simulink model "four_tanks_baseline"  (Simulink 7.5)
settings: Solver=ode45  StartTime=0.0  StopTime=8000  MaxStep=.25  RelTol=1e-3
model workspace (MAT data in the model file):
  gamma_1 : Simulink.Parameter (value not decoded)
  gamma_2 : Simulink.Parameter (value not decoded)
  a1 : Simulink.Parameter (value not decoded)
  a2 : Simulink.Parameter (value not decoded)
  a3 : Simulink.Parameter (value not decoded)
  a4 : Simulink.Parameter (value not decoded)
  g : Simulink.Parameter (value not decoded)
  A_1 : Simulink.Parameter (value not decoded)
  A_2 : Simulink.Parameter (value not decoded)
  A_3 : Simulink.Parameter (value not decoded)
  A_4 : Simulink.Parameter (value not decoded)
  x1o : Simulink.Parameter (value not decoded)
  x2o : Simulink.Parameter (value not decoded)
  x3o : Simulink.Parameter (value not decoded)
  x4o : Simulink.Parameter (value not decoded)
  x1_max : Simulink.Parameter (value not decoded)
  x2_max : Simulink.Parameter (value not decoded)
  x3_max : Simulink.Parameter (value not decoded)
  x4_max : Simulink.Parameter (value not decoded)
  u1_max : Simulink.Parameter (value not decoded)
  u2_max : Simulink.Parameter (value not decoded)
  x1f : Simulink.Parameter (value not decoded)
  x2f : Simulink.Parameter (value not decoded)
settings Model: Creator=Administrator  LastModifiedBy=jporter
settings DebuggingCC: StrictBusMsg=Warning

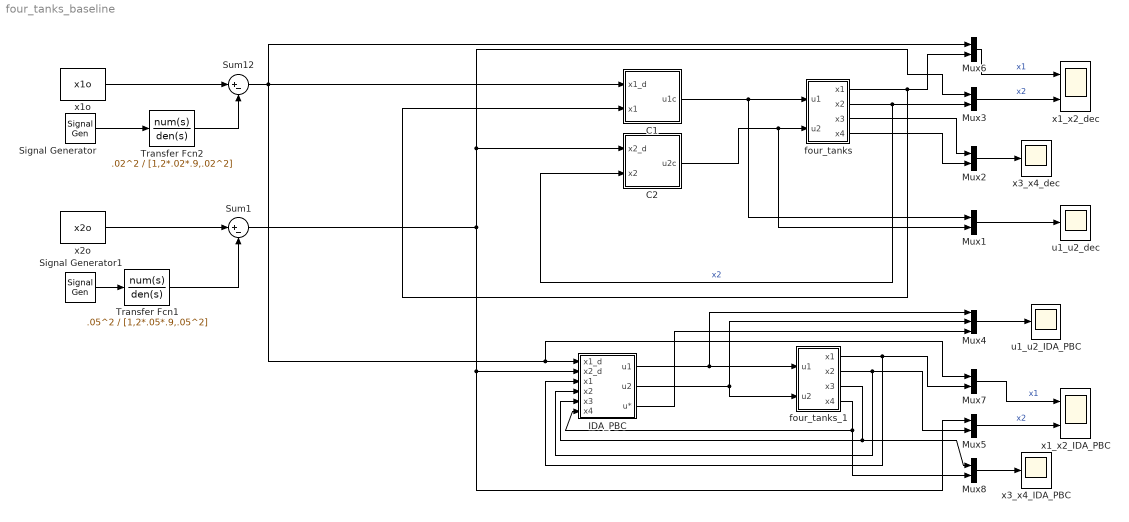
== system four_tanks_baseline ==
  C1 : Subsystem  mask{K=1.5, Ti=110, u1_max=100, gamma_1=gamma_1, gamma_2=gamma_2, x1o=x1o, x2o=x2o, a1=a1, a2=a2, g=g}
      mask prompts: u1_max "u1_max (ml/sec)"
      mask init:
      | L12 = [gamma_1, (1-gamma_2);
      |     (1-gamma_1),gamma_2];
      | us=inv(L12)*[a1*sqrt(2*g*x1o);a2*sqrt(2*g*x2o)];
      | xIo1=us(1)/K
  C2 : Subsystem  mask{K=-.12, Ti=220, u1_max=100, gamma_1=gamma_1, gamma_2=gamma_2, x1o=x1o, x2o=x2o, a1=a1, a2=a2, g=g}
      mask prompts: u1_max "u2_max (ml/sec)"
      mask init:
      | L12 = [gamma_1, (1-gamma_2);
      |     (1-gamma_1),gamma_2];
      | us=inv(L12)*[a1*sqrt(2*g*x1o);a2*sqrt(2*g*x2o)];
      | xIo2=us(2)/K
  IDA_PBC : Subsystem  mask{k1=.2, k2=.2, A_1=A_1, A_2=A_2, A_3=A_3, A_4=A_4, a1=a1, a2=a2, a3=a3, a4=a4, gamma_1=gamma_1, gamma_2=gamma_2, u1_max=u1_max, u2_max=u2_max, g=g}
      mask prompts: gamma_1 "gamma_1 in [0,1]"; gamma_2 "gamma_2 in [0,1]"; g "g (cm/s^2)"
      mask init:
      | k3=2*k1*A_3/(4*A_1);
      | k4=2*k2*A_4/(4*A_2);
      | kI1=0.1*(4-(k1/k3));
      | kI2=0.1*(4-(k2/k4));
      | JmR=[-1/(k1*A_1),0,1/(k3*A_1),0,0,0;
      |    0,-1/(k2*A_2),0,1/(k4*A_2),0,0;
      |    0,0,-1/(k3*A_3),0,0,0;
      |    0,0,0,-1/(k4*A_4),0,0;
      |    kI1/k1,0,0,0,-kI1/k1,0;
      |    0,kI2/k2,0,0,0,-kI2/k2];
      | eig(JmR)
      | P=[gamma_1*k1,(1-gamma_1)*k2,0,(1-gamma_1)*k4,gamma_1*k1,(1-gamma_1)*k2;
      |    (1-gamma_2)*k1,gamma_2*k2,(1-gamma_2)*k3,0,(1-gamma_2)*k1,gamma_2*k2];
      | L12=[gamma_1,(1-gamma_2);
      |     (1-gamma_1),gamma_2];
      | L34=[0,(1-gamma_2);
      |     (1-gamma_1),0];
      | Q=eye(2);
      | K=Q*P;
  Mux{1..3,5..8} (7 alike) : Mux  Inputs=2
  Mux4 : Mux  Inputs=[1,1,2]
  Signal Generator : SignalGenerator  WaveForm=square  Amplitude=x1f-x1o  Frequency=1/8000
  Signal Generator1 : SignalGenerator  WaveForm=square  Amplitude=x2f-x2o+.001  Frequency=1/8000
  Sum1 : Sum  Inputs=|+-  OutDataType=fixdt(1, 16)  OutScaling=2^0
  Sum12 : Sum  Inputs=|+-  OutDataType=fixdt(1, 16)  OutScaling=2^0
  Transfer Fcn1 : TransferFcn  Numerator=.05^2  Denominator=[1,2*.05*.9,.05^2]
  Transfer Fcn2 : TransferFcn  Numerator=.02^2  Denominator=[1,2*.02*.9,.02^2]
  four_tanks : Subsystem  mask{x1o=x1o, x2o=x2o, x3o=x3o, x4o=x4o, x1_max=x1_max, x2_max=x2_max, x3_max=x3_max, x4_max=x4_max, u1_max=100, u2_max=100, a1=a1, a2=a2, a3=a3, a4=a4, A_1=A_1, A_2=A_2, A_3=A_3, A_4=A_4, gamma_1=gamma_1, gamma_2=gamma_2, g=g}
      mask prompts: x1o "x1o (cm)"; x2o "x2o (cm)"; x3o "x3o (cm)"; x4o "x4o (cm)"; x1_max "x1_max (cm)"; x2_max "x2_max (cm)"; x3_max "x3_max (cm)"; x4_max "x4_max (cm)"; u1_max "u1_max (ml/s)"; u2_max "u2_max (ml/s)"; a1 "a1 (cm2)"; a2 "a2 (cm2)"; a3 "a3 (cm2)"; a4 "a4 (cm2)"; A_1 "A_1 (cm2)"; A_2 "A_2 (cm2)"; A_3 "A_3 (cm2)"; A_4 "A_4 (cm2)"; gamma_1 "gamma_1 in [0,1]"; gamma_2 "gamma_2 in [0,1]"; g "g (cm/s2)"
  four_tanks_1 : Subsystem  mask{x1o=x1o, x2o=x2o, x3o=x3o, x4o=x4o, x1_max=x1_max, x2_max=x2_max, x3_max=x3_max, x4_max=x4_max, u1_max=100, u2_max=100, a1=a1, a2=a2, a3=a3, a4=a4, A_1=A_1, A_2=A_2, A_3=A_3, A_4=A_4, gamma_1=gamma_1, gamma_2=gamma_2, g=g}
      mask prompts: x1o "x1o (cm)"; x2o "x2o (cm)"; x3o "x3o (cm)"; x4o "x4o (cm)"; x1_max "x1_max (cm)"; x2_max "x2_max (cm)"; x3_max "x3_max (cm)"; x4_max "x4_max (cm)"; u1_max "u1_max (ml/s)"; u2_max "u2_max (ml/s)"; a1 "a1 (cm2)"; a2 "a2 (cm2)"; a3 "a3 (cm2)"; a4 "a4 (cm2)"; A_1 "A_1 (cm2)"; A_2 "A_2 (cm2)"; A_3 "A_3 (cm2)"; A_4 "A_4 (cm2)"; gamma_1 "gamma_1 in [0,1]"; gamma_2 "gamma_2 in [0,1]"; g "g (cm/s2)"
  u1_u2_IDA_PBC : Scope
      settings: TimeRange=200  YMin=8.25  YMax=11  SampleInput=on  SampleTime=2
  u1_u2_dec : Scope
      settings: TimeRange=200  YMin=0  YMax=40  SaveName=ScopeData5  SampleInput=on  SampleTime=2
  x1_x2_IDA_PBC : Scope  NumInputPorts=2
      settings: YMin=7.5~7.5  YMax=17.5~17.5  SaveName=ScopeData2  SampleInput=on  SampleTime=2
  x1_x2_dec : Scope  NumInputPorts=2
      settings: YMin=1~2.5  YMax=15~15  SaveName=ScopeData6  SampleInput=on  SampleTime=2
  x1o : Constant  Value=x1o  OutDataType=fixdt(1, 16)  OutScaling=2^0
  x2o : Constant  Value=x2o  OutDataType=fixdt(1, 16)  OutScaling=2^0
  x3_x4_IDA_PBC : Scope
      settings: TimeRange=200  YMin=2  YMax=9.5  SaveName=ScopeData3  SampleInput=on  SampleTime=2
  x3_x4_dec : Scope
      settings: TimeRange=200  YMin=0  YMax=40  SampleInput=on  SampleTime=2
  wires:
  Signal Generator/1 -> Transfer Fcn2/1
  x1o/1 -> Sum12/1
  four_tanks/3(x3) -> Mux2/1
  four_tanks/4(x4) -> Mux2/2
  Mux1/1 -> u1_u2_dec/1
  Mux2/1 -> x3_x4_dec/1
  Sum12/1 -> IDA_PBC/1(x1_d), Mux7/1, Mux6/1, C1/1(x1_d)
  four_tanks/1(x1) -> C1/2(x1), Mux6/2
  four_tanks/2(x2) -> Mux3/2, C2/2(x2)  "x2"
  Transfer Fcn2/1 -> Sum12/2
  Mux3/1 -> x1_x2_dec/2  "x2"
  Mux6/1 -> x1_x2_dec/1  "x1"
  IDA_PBC/1(u1) -> four_tanks_1/1(u1), Mux4/1
  IDA_PBC/2(u2) -> four_tanks_1/2(u2), Mux4/2
  four_tanks_1/4(x4) -> IDA_PBC/6(x4), Mux8/2
  four_tanks_1/3(x3) -> IDA_PBC/5(x3), Mux8/1
  four_tanks_1/2(x2) -> IDA_PBC/4(x2), Mux5/2
  four_tanks_1/1(x1) -> IDA_PBC/3(x1), Mux7/2
  Mux4/1 -> u1_u2_IDA_PBC/1
  IDA_PBC/3(u*) -> Mux4/3
  Mux5/1 -> x1_x2_IDA_PBC/2  "x2"
  Mux7/1 -> x1_x2_IDA_PBC/1  "x1"
  Mux8/1 -> x3_x4_IDA_PBC/1
  Signal Generator1/1 -> Transfer Fcn1/1
  x2o/1 -> Sum1/1
  Transfer Fcn1/1 -> Sum1/2
  Sum1/1 -> IDA_PBC/2(x2_d), Mux5/1, Mux3/1, C2/1(x2_d)
  C1/1(u1c) -> four_tanks/1(u1), Mux1/1
  C2/1(u2c) -> four_tanks/2(u2), Mux1/2

== system four_tanks_baseline/C1 ==
  x1_d : Inport
  x1 : Inport  Port=2
  1/Ti : Gain  Gain=1/Ti  ParameterDataType=fixdt(1, 16)  ParameterScaling=2^0  OutDataType=fixdt(1, 16)  OutScaling=2^0
  Integrator1 : Integrator  InitialCondition=xIo1  LimitOutput=on  UpperSaturationLimit=u1_max/(abs(K))  LowerSaturationLimit=-u1_max/(abs(K))
  K : Gain  Gain=K  ParameterDataType=fixdt(1, 16)  ParameterScaling=2^0  OutDataType=fixdt(1, 16)  OutScaling=2^0
  SAT : Saturate  UpperLimit=u1_max  LowerLimit=0  OutDataType=fixdt(1, 16)  OutScaling=2^0
  Sum10 : Sum  Inputs=|+-  OutDataType=fixdt(1, 16)  OutScaling=2^0
  Sum11 : Sum  Inputs=++-  OutDataType=fixdt(1, 16)  OutScaling=2^0
  u1c : Outport
  wires:
  K/1 -> SAT/1
  Sum10/1 -> 1/Ti/1
  Sum11/1 -> K/1
  1/Ti/1 -> Integrator1/1
  Integrator1/1 -> Sum11/2
  x1_d/1 -> Sum11/1, Sum10/1
  SAT/1 -> u1c/1
  x1/1 -> Sum10/2, Sum11/3

== system four_tanks_baseline/C2 ==
  x2_d : Inport
  x2 : Inport  Port=2
  1/Ti : Gain  Gain=1/Ti  ParameterDataType=fixdt(1, 16)  ParameterScaling=2^0  OutDataType=fixdt(1, 16)  OutScaling=2^0
  Integrator1 : Integrator  InitialCondition=xIo2  LimitOutput=on  UpperSaturationLimit=u1_max/(abs(K))  LowerSaturationLimit=-u1_max/(abs(K))
  K : Gain  Gain=K  ParameterDataType=fixdt(1, 16)  ParameterScaling=2^0  OutDataType=fixdt(1, 16)  OutScaling=2^0
  SAT : Saturate  UpperLimit=u1_max  LowerLimit=0  OutDataType=fixdt(1, 16)  OutScaling=2^0
  Sum10 : Sum  Inputs=|+-  OutDataType=fixdt(1, 16)  OutScaling=2^0
  Sum11 : Sum  Inputs=++-  OutDataType=fixdt(1, 16)  OutScaling=2^0
  u2c : Outport
  wires:
  x2/1 -> Sum11/3, Sum10/2
  SAT/1 -> u2c/1
  x2_d/1 -> Sum10/1, Sum11/1
  Integrator1/1 -> Sum11/2
  1/Ti/1 -> Integrator1/1
  Sum11/1 -> K/1
  Sum10/1 -> 1/Ti/1
  K/1 -> SAT/1

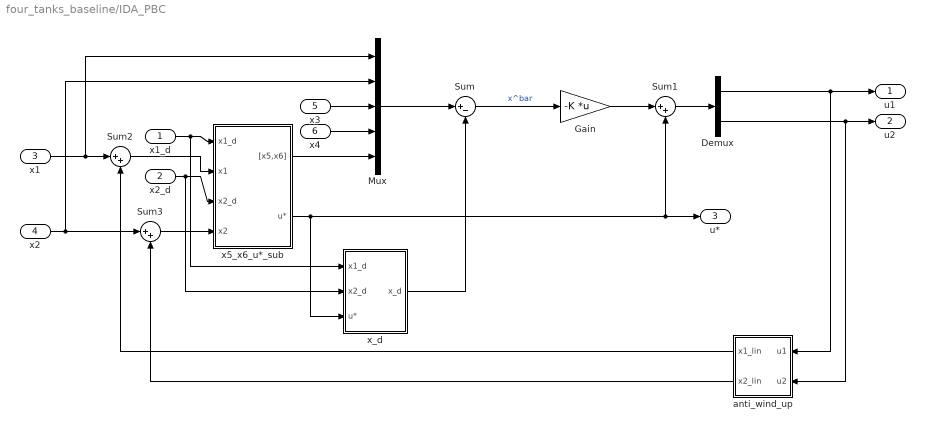
== system four_tanks_baseline/IDA_PBC ==
  x1_d : Inport
  x2_d : Inport  Port=2
  x1 : Inport  Port=3
  x2 : Inport  Port=4
  x3 : Inport  Port=5
  x4 : Inport  Port=6
  Demux : Demux  Outputs=2
  Gain : Gain  Gain=-K  Multiplication=Matrix(K*u)  ParameterDataType=fixdt(1, 16)  ParameterScaling=2^0  OutDataType=fixdt(1, 16)  OutScaling=2^0
  Mux : Mux  Inputs=[1,1,1,1,2]
  Sum : Sum  Inputs=|+-  OutDataType=fixdt(1, 16)  OutScaling=2^0
  Sum1 : Sum  Inputs=|++  OutDataType=fixdt(1, 16)  OutScaling=2^0
  Sum2 : Sum  Inputs=|++  OutDataType=fixdt(1, 16)  OutScaling=2^0
  Sum3 : Sum  Inputs=|++  OutDataType=fixdt(1, 16)  OutScaling=2^0
  anti_wind_up : Subsystem
  x5_x6_u*_sub : Subsystem
  x_d : Subsystem
  u1 : Outport
  u2 : Outport  Port=2
  u* : Outport  Port=3
  wires:
  x1_d/1 -> x5_x6_u*_sub/1(x1_d), x_d/1(x1_d)
  x1/1 -> Mux/1, Sum2/1
  x2_d/1 -> x5_x6_u*_sub/3(x2_d), x_d/2(x2_d)
  x2/1 -> Mux/2, Sum3/1
  x5_x6_u*_sub/1("[x5,x6]") -> Mux/5
  x3/1 -> Mux/3
  x4/1 -> Mux/4
  x5_x6_u*_sub/2(u*) -> x_d/3(u*), Sum1/2, u*/1
  Mux/1 -> Sum/1
  x_d/1(x_d) -> Sum/2
  Sum/1 -> Gain/1  "x^bar"
  Gain/1 -> Sum1/1
  Sum1/1 -> Demux/1
  Demux/1 -> u1/1, anti_wind_up/1(u1)
  Demux/2 -> u2/1, anti_wind_up/2(u2)
  anti_wind_up/1(x1_lin) -> Sum2/2
  Sum2/1 -> x5_x6_u*_sub/2(x1)
  Sum3/1 -> x5_x6_u*_sub/4(x2)
  anti_wind_up/2(x2_lin) -> Sum3/2

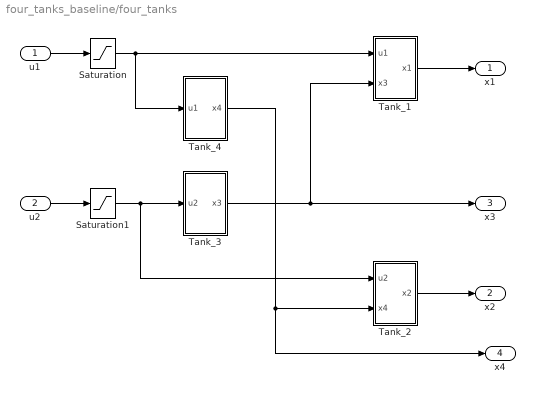
== system four_tanks_baseline/four_tanks ==
  u1 : Inport  OutDataType=fixdt(1, 16)  OutScaling=2^0
  u2 : Inport  Port=2  OutDataType=fixdt(1, 16)  OutScaling=2^0
  Saturation : Saturate  UpperLimit=u1_max  LowerLimit=0  OutDataType=fixdt(1, 16)  OutScaling=2^0
  Saturation1 : Saturate  UpperLimit=u2_max  LowerLimit=0  OutDataType=fixdt(1, 16)  OutScaling=2^0
  Tank_1 : Subsystem
  Tank_2 : Subsystem
  Tank_3 : Subsystem
  Tank_4 : Subsystem
  x1 : Outport  OutDataType=fixdt(1, 16)  OutScaling=2^0
  x2 : Outport  Port=2  OutDataType=fixdt(1, 16)  OutScaling=2^0
  x3 : Outport  Port=3  OutDataType=fixdt(1, 16)  OutScaling=2^0
  x4 : Outport  Port=4  OutDataType=fixdt(1, 16)  OutScaling=2^0
  wires:
  u1/1 -> Saturation/1
  Tank_1/1(x1) -> x1/1
  Tank_2/1(x2) -> x2/1
  u2/1 -> Saturation1/1
  Saturation/1 -> Tank_1/1(u1), Tank_4/1(u1)
  Saturation1/1 -> Tank_3/1(u2), Tank_2/1(u2)
  Tank_3/1(x3) -> Tank_1/2(x3), x3/1
  Tank_4/1(x4) -> Tank_2/2(x4), x4/1

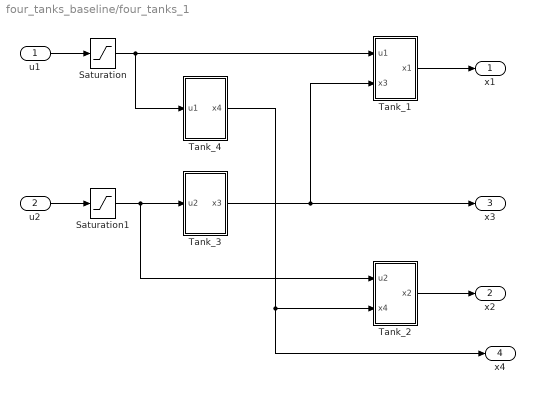
== system four_tanks_baseline/four_tanks_1 ==
  u1 : Inport  OutDataType=fixdt(1, 16)  OutScaling=2^0
  u2 : Inport  Port=2  OutDataType=fixdt(1, 16)  OutScaling=2^0
  Saturation : Saturate  UpperLimit=u1_max  LowerLimit=0  OutDataType=fixdt(1, 16)  OutScaling=2^0
  Saturation1 : Saturate  UpperLimit=u2_max  LowerLimit=0  OutDataType=fixdt(1, 16)  OutScaling=2^0
  Tank_1 : Subsystem
  Tank_2 : Subsystem
  Tank_3 : Subsystem
  Tank_4 : Subsystem
  x1 : Outport  OutDataType=fixdt(1, 16)  OutScaling=2^0
  x2 : Outport  Port=2  OutDataType=fixdt(1, 16)  OutScaling=2^0
  x3 : Outport  Port=3  OutDataType=fixdt(1, 16)  OutScaling=2^0
  x4 : Outport  Port=4  OutDataType=fixdt(1, 16)  OutScaling=2^0
  wires:
  Tank_4/1(x4) -> x4/1, Tank_2/2(x4)
  Tank_3/1(x3) -> x3/1, Tank_1/2(x3)
  Saturation1/1 -> Tank_2/1(u2), Tank_3/1(u2)
  Saturation/1 -> Tank_4/1(u1), Tank_1/1(u1)
  u2/1 -> Saturation1/1
  Tank_2/1(x2) -> x2/1
  Tank_1/1(x1) -> x1/1
  u1/1 -> Saturation/1

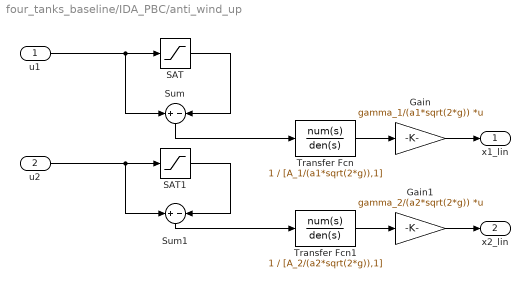
== system four_tanks_baseline/IDA_PBC/anti_wind_up ==
  u1 : Inport
  u2 : Inport  Port=2
  Gain : Gain  Gain=gamma_1/(a1*sqrt(2*g))  Multiplication=Matrix(K*u)  ParameterDataType=fixdt(1, 16)  ParameterScaling=2^0  OutDataType=fixdt(1, 16)  OutScaling=2^0
  Gain1 : Gain  Gain=gamma_2/(a2*sqrt(2*g))  Multiplication=Matrix(K*u)  ParameterDataType=fixdt(1, 16)  ParameterScaling=2^0  OutDataType=fixdt(1, 16)  OutScaling=2^0
  SAT : Saturate  UpperLimit=u1_max  LowerLimit=0  OutDataType=fixdt(1, 16)  OutScaling=2^0
  SAT1 : Saturate  UpperLimit=u1_max  LowerLimit=0  OutDataType=fixdt(1, 16)  OutScaling=2^0
  Sum : Sum  Inputs=+-  OutDataType=fixdt(1, 16)  OutScaling=2^0
  Sum1 : Sum  Inputs=+-  OutDataType=fixdt(1, 16)  OutScaling=2^0
  Transfer Fcn : TransferFcn  Numerator=1  Denominator=[A_1/(a1*sqrt(2*g)),1]
  Transfer Fcn1 : TransferFcn  Numerator=1  Denominator=[A_2/(a2*sqrt(2*g)),1]
  x1_lin : Outport
  x2_lin : Outport  Port=2
  wires:
  u1/1 -> SAT/1, Sum/1
  u2/1 -> SAT1/1, Sum1/1
  SAT/1 -> Sum/2
  SAT1/1 -> Sum1/2
  Sum/1 -> Transfer Fcn/1
  Transfer Fcn/1 -> Gain/1
  Gain/1 -> x1_lin/1
  Transfer Fcn1/1 -> Gain1/1
  Gain1/1 -> x2_lin/1
  Sum1/1 -> Transfer Fcn1/1

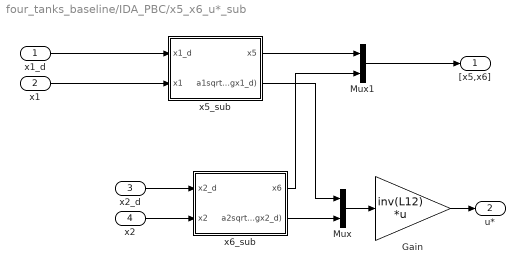
== system four_tanks_baseline/IDA_PBC/x5_x6_u*_sub ==
  x1_d : Inport
  x1 : Inport  Port=2
  x2_d : Inport  Port=3
  x2 : Inport  Port=4
  Gain : Gain  Gain=inv(L12)  Multiplication=Matrix(K*u)  ParameterDataType=fixdt(1, 16)  ParameterScaling=2^0  OutDataType=fixdt(1, 16)  OutScaling=2^0
  Mux : Mux  Inputs=2
  Mux1 : Mux  Inputs=2
  x5_sub : Subsystem
  x6_sub : Subsystem
  "[x5,x6]" : Outport
  u* : Outport  Port=2
  wires:
  x5_sub/2(a1sqrt(2gx1_d)) -> Mux/1
  x6_sub/2(a2sqrt(2gx2_d)) -> Mux/2
  Mux/1 -> Gain/1
  x5_sub/1(x5) -> Mux1/1
  x6_sub/1(x6) -> Mux1/2
  x1_d/1 -> x5_sub/1(x1_d)
  Mux1/1 -> "[x5,x6]"/1
  x1/1 -> x5_sub/2(x1)
  x2_d/1 -> x6_sub/1(x2_d)
  x2/1 -> x6_sub/2(x2)
  Gain/1 -> u*/1

== system four_tanks_baseline/IDA_PBC/x_d ==
  x1_d : Inport
  x2_d : Inport  Port=2
  u* : Inport  Port=3
  Mux1 : Mux  Inputs=[1,1,2,2]
  gen_x3d_x4d : Subsystem
  x5d_x6d : Constant  Value=[0,0]  OutDataType=fixdt(1, 16)  OutScaling=2^0
  x_d : Outport
  wires:
  x5d_x6d/1 -> Mux1/4
  gen_x3d_x4d/1("[x3d,x4d]") -> Mux1/3
  x1_d/1 -> Mux1/1
  x2_d/1 -> Mux1/2
  Mux1/1 -> x_d/1
  u*/1 -> gen_x3d_x4d/1(u*)

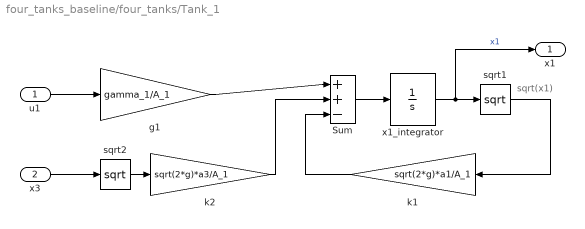
== system four_tanks_baseline/four_tanks/Tank_1 ==
  note: sqrt(x1)
  u1 : Inport
  x3 : Inport  Port=2
  Sum : Sum  Inputs=|++-  OutDataType=fixdt(1, 16)  OutScaling=2^0
  g1 : Gain  Gain=gamma_1/A_1  ParameterDataType=fixdt(1, 16)  ParameterScaling=2^0  OutDataType=fixdt(1, 16)  OutScaling=2^0
  k1 : Gain  Gain=sqrt(2*g)*a1/A_1  ParameterDataType=fixdt(1, 16)  ParameterScaling=2^0  OutDataType=fixdt(1, 16)  OutScaling=2^0
  k2 : Gain  Gain=sqrt(2*g)*a3/A_1  ParameterDataType=fixdt(1, 16)  ParameterScaling=2^0  OutDataType=fixdt(1, 16)  OutScaling=2^0
  sqrt1 : Math  Operator=sqrt  OutDataType=fixdt(1, 16)  OutScaling=2^0  SaturateOnIntegerOverflow=on
  sqrt2 : Math  Operator=sqrt  OutDataType=fixdt(1, 16)  OutScaling=2^0  SaturateOnIntegerOverflow=on
  x1_integrator : Integrator  InitialCondition=x1o  LimitOutput=on  UpperSaturationLimit=x1_max  LowerSaturationLimit=0
  x1 : Outport
  wires:
  g1/1 -> Sum/1
  x1_integrator/1 -> sqrt1/1, x1/1  "x1"
  sqrt1/1 -> k1/1
  k1/1 -> Sum/3
  Sum/1 -> x1_integrator/1
  u1/1 -> g1/1
  x3/1 -> sqrt2/1
  sqrt2/1 -> k2/1
  k2/1 -> Sum/2

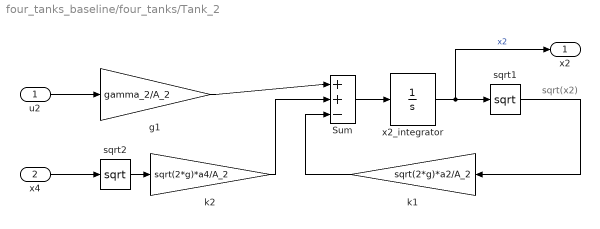
== system four_tanks_baseline/four_tanks/Tank_2 ==
  note: sqrt(x2)
  u2 : Inport
  x4 : Inport  Port=2
  Sum : Sum  Inputs=|++-  OutDataType=fixdt(1, 16)  OutScaling=2^0
  g1 : Gain  Gain=gamma_2/A_2  ParameterDataType=fixdt(1, 16)  ParameterScaling=2^0  OutDataType=fixdt(1, 16)  OutScaling=2^0
  k1 : Gain  Gain=sqrt(2*g)*a2/A_2  ParameterDataType=fixdt(1, 16)  ParameterScaling=2^0  OutDataType=fixdt(1, 16)  OutScaling=2^0
  k2 : Gain  Gain=sqrt(2*g)*a4/A_2  ParameterDataType=fixdt(1, 16)  ParameterScaling=2^0  OutDataType=fixdt(1, 16)  OutScaling=2^0
  sqrt1 : Math  Operator=sqrt  OutDataType=fixdt(1, 16)  OutScaling=2^0  SaturateOnIntegerOverflow=on
  sqrt2 : Math  Operator=sqrt  OutDataType=fixdt(1, 16)  OutScaling=2^0  SaturateOnIntegerOverflow=on
  x2_integrator : Integrator  InitialCondition=x2o  LimitOutput=on  UpperSaturationLimit=x2_max  LowerSaturationLimit=0
  x2 : Outport
  wires:
  k2/1 -> Sum/2
  sqrt2/1 -> k2/1
  x4/1 -> sqrt2/1
  u2/1 -> g1/1
  Sum/1 -> x2_integrator/1
  k1/1 -> Sum/3
  sqrt1/1 -> k1/1
  x2_integrator/1 -> x2/1, sqrt1/1  "x2"
  g1/1 -> Sum/1

== system four_tanks_baseline/four_tanks/Tank_3 ==
  note: sqrt(x3)
  u2 : Inport
  Sum : Sum  Inputs=|+-  OutDataType=fixdt(1, 16)  OutScaling=2^0
  g1 : Gain  Gain=(1-gamma_2)/A_3  ParameterDataType=fixdt(1, 16)  ParameterScaling=2^0  OutDataType=fixdt(1, 16)  OutScaling=2^0
  k1 : Gain  Gain=sqrt(2*g)*a3/A_3  ParameterDataType=fixdt(1, 16)  ParameterScaling=2^0  OutDataType=fixdt(1, 16)  OutScaling=2^0
  sqrt1 : Math  Operator=sqrt  OutDataType=fixdt(1, 16)  OutScaling=2^0  SaturateOnIntegerOverflow=on
  x3_integrator : Integrator  InitialCondition=x3o  LimitOutput=on  UpperSaturationLimit=x3_max  LowerSaturationLimit=0
  x3 : Outport
  wires:
  g1/1 -> Sum/1
  x3_integrator/1 -> sqrt1/1, x3/1  "x3"
  sqrt1/1 -> k1/1
  Sum/1 -> x3_integrator/1
  u2/1 -> g1/1
  k1/1 -> Sum/2

== system four_tanks_baseline/four_tanks/Tank_4 ==
  note: sqrt(x4)
  u1 : Inport
  Sum : Sum  Inputs=|+-  OutDataType=fixdt(1, 16)  OutScaling=2^0
  g1 : Gain  Gain=(1-gamma_1)/A_4  ParameterDataType=fixdt(1, 16)  ParameterScaling=2^0  OutDataType=fixdt(1, 16)  OutScaling=2^0
  k1 : Gain  Gain=sqrt(2*g)*a4/A_4  ParameterDataType=fixdt(1, 16)  ParameterScaling=2^0  OutDataType=fixdt(1, 16)  OutScaling=2^0
  sqrt1 : Math  Operator=sqrt  OutDataType=fixdt(1, 16)  OutScaling=2^0  SaturateOnIntegerOverflow=on
  x4_integrator : Integrator  InitialCondition=x4o  LimitOutput=on  UpperSaturationLimit=x4_max  LowerSaturationLimit=0
  x4 : Outport
  wires:
  k1/1 -> Sum/2
  u1/1 -> g1/1
  Sum/1 -> x4_integrator/1
  sqrt1/1 -> k1/1
  x4_integrator/1 -> x4/1, sqrt1/1  "x4"
  g1/1 -> Sum/1

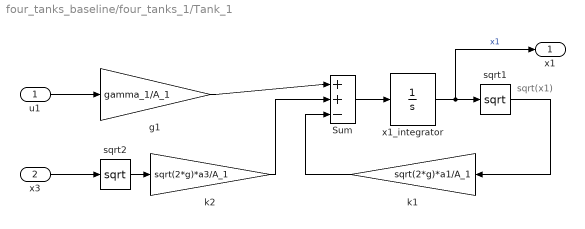
== system four_tanks_baseline/four_tanks_1/Tank_1 ==
  note: sqrt(x1)
  u1 : Inport
  x3 : Inport  Port=2
  Sum : Sum  Inputs=|++-  OutDataType=fixdt(1, 16)  OutScaling=2^0
  g1 : Gain  Gain=gamma_1/A_1  ParameterDataType=fixdt(1, 16)  ParameterScaling=2^0  OutDataType=fixdt(1, 16)  OutScaling=2^0
  k1 : Gain  Gain=sqrt(2*g)*a1/A_1  ParameterDataType=fixdt(1, 16)  ParameterScaling=2^0  OutDataType=fixdt(1, 16)  OutScaling=2^0
  k2 : Gain  Gain=sqrt(2*g)*a3/A_1  ParameterDataType=fixdt(1, 16)  ParameterScaling=2^0  OutDataType=fixdt(1, 16)  OutScaling=2^0
  sqrt1 : Math  Operator=sqrt  OutDataType=fixdt(1, 16)  OutScaling=2^0  SaturateOnIntegerOverflow=on
  sqrt2 : Math  Operator=sqrt  OutDataType=fixdt(1, 16)  OutScaling=2^0  SaturateOnIntegerOverflow=on
  x1_integrator : Integrator  InitialCondition=x1o  LimitOutput=on  UpperSaturationLimit=x1_max  LowerSaturationLimit=0
  x1 : Outport
  wires:
  k2/1 -> Sum/2
  sqrt2/1 -> k2/1
  x3/1 -> sqrt2/1
  u1/1 -> g1/1
  Sum/1 -> x1_integrator/1
  k1/1 -> Sum/3
  sqrt1/1 -> k1/1
  x1_integrator/1 -> x1/1, sqrt1/1  "x1"
  g1/1 -> Sum/1

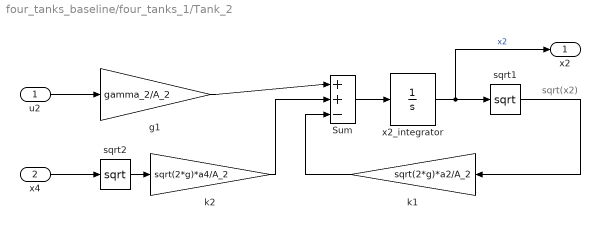
== system four_tanks_baseline/four_tanks_1/Tank_2 ==
  note: sqrt(x2)
  u2 : Inport
  x4 : Inport  Port=2
  Sum : Sum  Inputs=|++-  OutDataType=fixdt(1, 16)  OutScaling=2^0
  g1 : Gain  Gain=gamma_2/A_2  ParameterDataType=fixdt(1, 16)  ParameterScaling=2^0  OutDataType=fixdt(1, 16)  OutScaling=2^0
  k1 : Gain  Gain=sqrt(2*g)*a2/A_2  ParameterDataType=fixdt(1, 16)  ParameterScaling=2^0  OutDataType=fixdt(1, 16)  OutScaling=2^0
  k2 : Gain  Gain=sqrt(2*g)*a4/A_2  ParameterDataType=fixdt(1, 16)  ParameterScaling=2^0  OutDataType=fixdt(1, 16)  OutScaling=2^0
  sqrt1 : Math  Operator=sqrt  OutDataType=fixdt(1, 16)  OutScaling=2^0  SaturateOnIntegerOverflow=on
  sqrt2 : Math  Operator=sqrt  OutDataType=fixdt(1, 16)  OutScaling=2^0  SaturateOnIntegerOverflow=on
  x2_integrator : Integrator  InitialCondition=x2o  LimitOutput=on  UpperSaturationLimit=x2_max  LowerSaturationLimit=0
  x2 : Outport
  wires:
  g1/1 -> Sum/1
  x2_integrator/1 -> sqrt1/1, x2/1  "x2"
  sqrt1/1 -> k1/1
  k1/1 -> Sum/3
  Sum/1 -> x2_integrator/1
  u2/1 -> g1/1
  x4/1 -> sqrt2/1
  sqrt2/1 -> k2/1
  k2/1 -> Sum/2

== system four_tanks_baseline/four_tanks_1/Tank_3 ==
  note: sqrt(x3)
  u2 : Inport
  Sum : Sum  Inputs=|+-  OutDataType=fixdt(1, 16)  OutScaling=2^0
  g1 : Gain  Gain=(1-gamma_2)/A_3  ParameterDataType=fixdt(1, 16)  ParameterScaling=2^0  OutDataType=fixdt(1, 16)  OutScaling=2^0
  k1 : Gain  Gain=sqrt(2*g)*a3/A_3  ParameterDataType=fixdt(1, 16)  ParameterScaling=2^0  OutDataType=fixdt(1, 16)  OutScaling=2^0
  sqrt1 : Math  Operator=sqrt  OutDataType=fixdt(1, 16)  OutScaling=2^0  SaturateOnIntegerOverflow=on
  x3_integrator : Integrator  InitialCondition=x3o  LimitOutput=on  UpperSaturationLimit=x3_max  LowerSaturationLimit=0
  x3 : Outport
  wires:
  k1/1 -> Sum/2
  u2/1 -> g1/1
  Sum/1 -> x3_integrator/1
  sqrt1/1 -> k1/1
  x3_integrator/1 -> x3/1, sqrt1/1  "x3"
  g1/1 -> Sum/1

== system four_tanks_baseline/four_tanks_1/Tank_4 ==
  note: sqrt(x4)
  u1 : Inport
  Sum : Sum  Inputs=|+-  OutDataType=fixdt(1, 16)  OutScaling=2^0
  g1 : Gain  Gain=(1-gamma_1)/A_4  ParameterDataType=fixdt(1, 16)  ParameterScaling=2^0  OutDataType=fixdt(1, 16)  OutScaling=2^0
  k1 : Gain  Gain=sqrt(2*g)*a4/A_4  ParameterDataType=fixdt(1, 16)  ParameterScaling=2^0  OutDataType=fixdt(1, 16)  OutScaling=2^0
  sqrt1 : Math  Operator=sqrt  OutDataType=fixdt(1, 16)  OutScaling=2^0  SaturateOnIntegerOverflow=on
  x4_integrator : Integrator  InitialCondition=x4o  LimitOutput=on  UpperSaturationLimit=x4_max  LowerSaturationLimit=0
  x4 : Outport
  wires:
  g1/1 -> Sum/1
  x4_integrator/1 -> sqrt1/1, x4/1  "x4"
  sqrt1/1 -> k1/1
  Sum/1 -> x4_integrator/1
  u1/1 -> g1/1
  k1/1 -> Sum/2

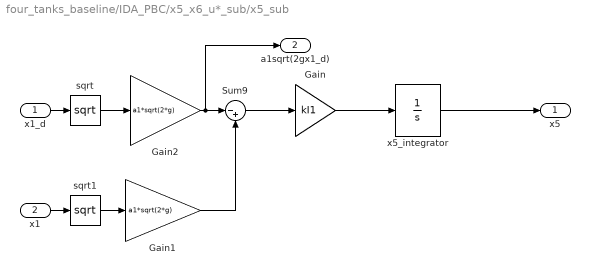
== system four_tanks_baseline/IDA_PBC/x5_x6_u*_sub/x5_sub ==
  x1_d : Inport
  x1 : Inport  Port=2
  Gain : Gain  Gain=kI1  ParameterDataType=fixdt(1, 16)  ParameterScaling=2^0  OutDataType=fixdt(1, 16)  OutScaling=2^0
  Gain1 : Gain  Gain=a1*sqrt(2*g)  ParameterDataType=fixdt(1, 16)  ParameterScaling=2^0  OutDataType=fixdt(1, 16)  OutScaling=2^0
  Gain2 : Gain  Gain=a1*sqrt(2*g)  ParameterDataType=fixdt(1, 16)  ParameterScaling=2^0  OutDataType=fixdt(1, 16)  OutScaling=2^0
  Sum9 : Sum  Inputs=|-+  OutDataType=fixdt(1, 16)  OutScaling=2^0
  sqrt : Math  Operator=sqrt  OutDataType=fixdt(1, 16)  OutScaling=2^0  SaturateOnIntegerOverflow=on
  sqrt1 : Math  Operator=sqrt  OutDataType=fixdt(1, 16)  OutScaling=2^0  SaturateOnIntegerOverflow=on
  x5_integrator : Integrator  UpperSaturationLimit=.1*sqrt(2*g*100)  LowerSaturationLimit=-.1*sqrt(2*g*100)
  x5 : Outport
  a1sqrt(2gx1_d) : Outport  Port=2
  wires:
  sqrt/1 -> Gain2/1
  sqrt1/1 -> Gain1/1
  Sum9/1 -> Gain/1
  x1_d/1 -> sqrt/1
  x5_integrator/1 -> x5/1
  x1/1 -> sqrt1/1
  Gain1/1 -> Sum9/2
  Gain2/1 -> Sum9/1, a1sqrt(2gx1_d)/1
  Gain/1 -> x5_integrator/1

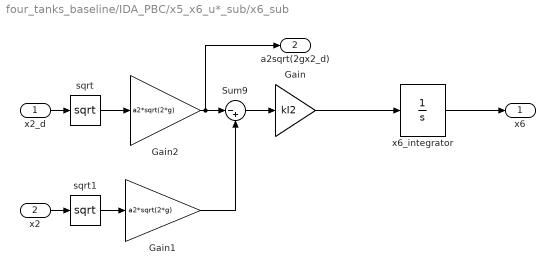
== system four_tanks_baseline/IDA_PBC/x5_x6_u*_sub/x6_sub ==
  x2_d : Inport
  x2 : Inport  Port=2
  Gain : Gain  Gain=kI2  ParameterDataType=fixdt(1, 16)  ParameterScaling=2^0  OutDataType=fixdt(1, 16)  OutScaling=2^0
  Gain1 : Gain  Gain=a2*sqrt(2*g)  ParameterDataType=fixdt(1, 16)  ParameterScaling=2^0  OutDataType=fixdt(1, 16)  OutScaling=2^0
  Gain2 : Gain  Gain=a2*sqrt(2*g)  ParameterDataType=fixdt(1, 16)  ParameterScaling=2^0  OutDataType=fixdt(1, 16)  OutScaling=2^0
  Sum9 : Sum  Inputs=|-+  OutDataType=fixdt(1, 16)  OutScaling=2^0
  sqrt : Math  Operator=sqrt  OutDataType=fixdt(1, 16)  OutScaling=2^0  SaturateOnIntegerOverflow=on
  sqrt1 : Math  Operator=sqrt  OutDataType=fixdt(1, 16)  OutScaling=2^0  SaturateOnIntegerOverflow=on
  x6_integrator : Integrator  UpperSaturationLimit=.1*sqrt(2*g*100)  LowerSaturationLimit=-.1*sqrt(2*g*100)
  x6 : Outport
  a2sqrt(2gx2_d) : Outport  Port=2
  wires:
  Gain2/1 -> a2sqrt(2gx2_d)/1, Sum9/1
  Gain1/1 -> Sum9/2
  x2/1 -> sqrt1/1
  x6_integrator/1 -> x6/1
  x2_d/1 -> sqrt/1
  Sum9/1 -> Gain/1
  sqrt1/1 -> Gain1/1
  sqrt/1 -> Gain2/1
  Gain/1 -> x6_integrator/1

== system four_tanks_baseline/IDA_PBC/x_d/gen_x3d_x4d ==
  u* : Inport
  L1 : Gain  Gain=1/(2*g)  ParameterDataType=fixdt(1, 16)  ParameterScaling=2^0  OutDataType=fixdt(1, 16)  OutScaling=2^0
  L34 : Gain  Gain=L34  Multiplication=Matrix(K*u)  ParameterDataType=fixdt(1, 16)  ParameterScaling=2^0  OutDataType=fixdt(1, 16)  OutScaling=2^0
  Product : Product  OutDataType=fixdt(1, 16)  OutScaling=2^0  RndMeth=Zero
  scale : Gain  Gain=[1/a3,0;0,1/a4]  Multiplication=Matrix(K*u)  ParameterDataType=fixdt(1, 16)  ParameterScaling=2^0  OutDataType=fixdt(1, 16)  OutScaling=2^0
  "[x3d,x4d]" : Outport
  wires:
  L34/1 -> scale/1
  scale/1 -> Product/2, Product/1
  Product/1 -> L1/1
  L1/1 -> "[x3d,x4d]"/1
  u*/1 -> L34/1
